simulink model "simulink_punto7_nonlineare_2"  (R2025b)
settings: Solver=VariableStepAuto  StartTime=0.0  StopTime=10.0  RelTol=1e-3
values from neighbouring files (symbols this model uses):
  A_7_2 = [0 1 0 0 0 ... (first row only)    [CODE_42_01.m]    (also in nonlinear_analisys_and_simulation.m)
  alpha_0 = invpendulumP.alpha_0    [CODE_42_01.m]    (also in nonlinear_analisys_and_simulation.m)
  alpha_1 = invpendulumP.alpha_1    [CODE_42_01.m]    (also in nonlinear_analisys_and_simulation.m)
  b = invpendulumP.b    [CODE_42_01.m]    (also in nonlinear_analisys_and_simulation.m)
  B_7_2 = [0,0 ... (first row only)    [CODE_42_01.m]    (also in nonlinear_analisys_and_simulation.m)
  c = invpendulumP.c    [CODE_42_01.m]    (also in nonlinear_analisys_and_simulation.m)
  C_7 = [1 0 0 0 0 ... (first row only)    [CODE_42_01.m]    (also in nonlinear_analisys_and_simulation.m)
  g = invpendulumP.g    [CODE_42_01.m]    (also in nonlinear_analisys_and_simulation.m)
  I_0 = invpendulumP.I_0    [CODE_42_01.m]    (also in nonlinear_analisys_and_simulation.m)
  I_1 = invpendulumP.I_1    [CODE_42_01.m]    (also in nonlinear_analisys_and_simulation.m)
  I_2 = invpendulumP.I_2    [CODE_42_01.m]    (also in nonlinear_analisys_and_simulation.m)
  K2 = place(A_7_2, B_7_2(:,1), pC2)    [CODE_42_01.m]    (also in nonlinear_analisys_and_simulation.m)
  kt = invpendulumP.kt    [CODE_42_01.m]    (also in nonlinear_analisys_and_simulation.m)
  L2 = 0.1    [CODE_42_01.m]    (also in nonlinear_analisys_and_simulation.m = 0.76)
  L_27 = lT_o_27'    [CODE_42_01.m]    (also in nonlinear_analisys_and_simulation.m)
  M = invpendulumP.M    [CODE_42_01.m]    (also in nonlinear_analisys_and_simulation.m)
  R = 1    [CODE_42_01.m]    (also in nonlinear_analisys_and_simulation.m = 3.6)
  r = invpendulumP.r    [CODE_42_01.m]    (also in nonlinear_analisys_and_simulation.m)
settings Model: Creator=palla  LastModifiedBy=palla

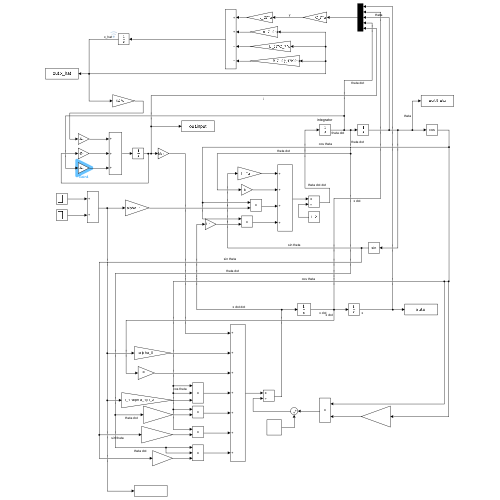
[thumbnail: Simulink's stored preview of the top-level diagram]
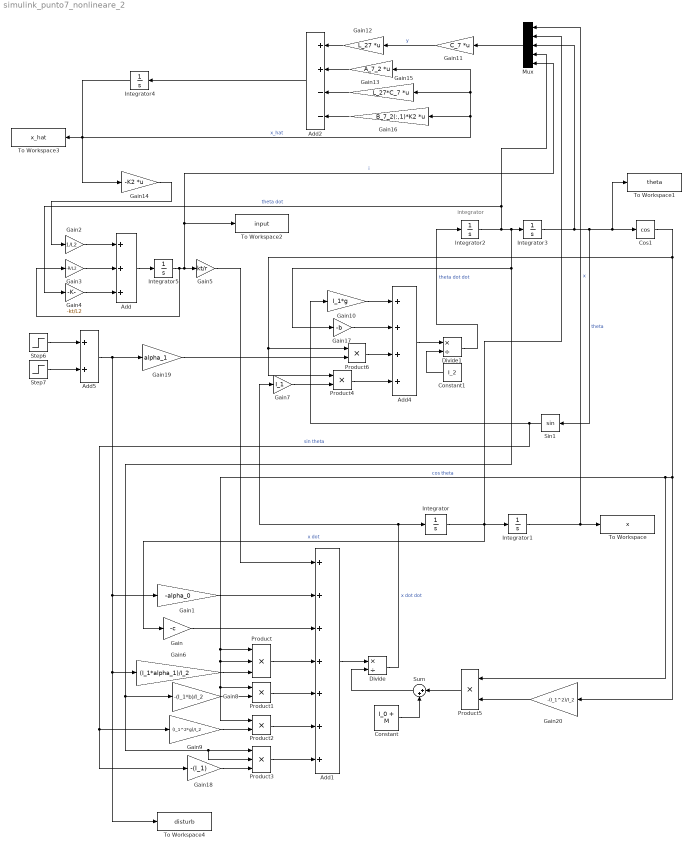
== system simulink_punto7_nonlineare_2 ==
  note: integrator
  Add : Sum  Inputs=+++
  Add1 : Sum  Inputs=+++++++
  Add2 : Sum  Inputs=++--
  Add4 : Sum  Inputs=++++
  Add5 : Sum
  Constant : Constant  Value=I_0 + M
  Constant1 : Constant  Value=I_2
  Cos1 : Trigonometry  Operator=cos
  Divide : Product  Inputs=*/
  Divide1 : Product  Inputs=*/
  Gain : Gain  Gain=-c
  Gain1 : Gain  Gain=-alpha_0
  Gain10 : Gain  Gain=I_1*g
  Gain11 : Gain  Gain=C_7  Multiplication=Matrix(K*u)
  Gain12 : Gain  Gain=L_27  Multiplication=Matrix(K*u)
  Gain13 : Gain  Gain=A_7_2  Multiplication=Matrix(K*u)
  Gain14 : Gain  Gain=-K2  Multiplication=Matrix(K*u)
  Gain15 : Gain  Gain=L_27*C_7  Multiplication=Matrix(K*u)
  Gain16 : Gain  Gain=B_7_2(:,1)*K2  Multiplication=Matrix(K*u)
  Gain17 : Gain  Gain=-b
  Gain18 : Gain  Gain=-(I_1)
  Gain19 : Gain  Gain=alpha_1
  Gain2 : Gain  Gain=1/L2
  Gain20 : Gain  Gain=-(I_1^2)/I_2
  Gain3 : Gain  Gain=-R/L2
  Gain4 : Gain  Gain=-kt/L2
  Gain5 : Gain  Gain=kt/r
  Gain6 : Gain  Gain=(I_1*alpha_1)/I_2
  Gain7 : Gain  Gain=I_1
  Gain8 : Gain  Gain=-(I_1*b)/I_2
  Gain9 : Gain  Gain=(I_1^2*g)/I_2
  Integrator{,1..3,5} (5 alike) : Integrator
  Integrator4 : Integrator  InitialCondition=zeros(5,1)
  Mux : Mux  Inputs=5
  Product : Product  Inputs=3
  Product{1..2,4..6} (5 alike) : Product
  Product3 : Product  Inputs=3
  Sin1 : Trigonometry
  Step6 : Step  SampleTime=0
  Step7 : Step  Time=3  After=-1  SampleTime=0
  Sum : Sum  Inputs=|++
  To Workspace : ToWorkspace  VariableName=x  SampleTime=-1
  To Workspace1 : ToWorkspace  VariableName=theta  SampleTime=-1
  To Workspace2 : ToWorkspace  VariableName=input  SampleTime=-1
  To Workspace3 : ToWorkspace  VariableName=x_hat  SampleTime=-1
  To Workspace4 : ToWorkspace  VariableName=disturb  SaveFormat=Timeseries  SampleTime=-1
  wires:
  Gain2/1 -> Add/1
  Add/1 -> Integrator5/1
  Gain4/1 -> Add/3
  Gain3/1 -> Add/2
  Integrator1/1 -> Mux/1, To Workspace/1  "x"
  Mux/1 -> Gain11/1
  Product6/1 -> Add4/3
  Add1/1 -> Divide/1
  Gain1/1 -> Add1/2
  Product1/1 -> Add1/5
  Gain/1 -> Add1/3
  Gain18/1 -> Product3/3
  Sin1/1 -> Gain10/1, Gain9/1, Gain18/1  "sin theta"
  Product/1 -> Add1/4
  Integrator2/1 -> Mux/4, Gain4/1, Gain17/1, Gain8/1, Product3/2, Product3/1, Integrator3/1  "theta dot"
  Gain7/1 -> Product4/2
  Product2/1 -> Add1/6
  Divide/1 -> Gain7/1, Integrator/1  "x dot dot"
  Constant1/1 -> Divide1/2
  Gain11/1 -> Gain12/1  "y"
  Gain20/1 -> Product5/2
  Gain10/1 -> Add4/1
  Step6/1 -> Add5/1
  Constant/1 -> Sum/2
  Cos1/1 -> Product/1, Product/2, Product1/1, Product2/1, Product5/1, Gain20/1, Product6/1, Product4/1  "cos theta"
  Integrator4/1 -> Gain14/1, Gain16/1, Gain15/1, Gain13/1, To Workspace3/1  "x_hat"
  Gain13/1 -> Add2/2
  Gain17/1 -> Add4/2
  Step7/1 -> Add5/2
  Divide1/1 -> Integrator2/1  "theta dot dot"
  Gain16/1 -> Add2/4
  Add5/1 -> Gain6/1, To Workspace4/1, Gain1/1, Gain19/1
  Gain6/1 -> Product/3
  Sum/1 -> Divide/2
  Gain8/1 -> Product1/2
  Gain12/1 -> Add2/1
  Gain9/1 -> Product2/2
  Add4/1 -> Divide1/1
  Product4/1 -> Add4/4
  Integrator/1 -> Mux/2, Gain/1, Integrator1/1  "x dot"
  Product3/1 -> Add1/7
  Integrator3/1 -> Mux/3, To Workspace1/1, Cos1/1, Sin1/1  "theta"
  Gain15/1 -> Add2/3
  Gain19/1 -> Product6/2
  Product5/1 -> Sum/1
  Gain14/1 -> Gain2/1
  Integrator5/1 -> Gain3/1, Mux/5, To Workspace2/1, Gain5/1  "i"
  Gain5/1 -> Add1/1
  Add2/1 -> Integrator4/1
